simulink model "psbrectifier"  (Simulink 6.0)
settings: Solver=ode23tb  SolverMode=SingleTasking  StartTime=0.0  StopTime=0.1  RelTol=1e-3
libraries: powerlib2 x20
settings Model: Creator=patrice  LastModifiedBy=batserve  ExtModeTrigMode=oneshot  ExtModeArmWhenConnect=off  ExtModeAutoUpdateStatusClock=off
settings DataIOCC: LimitDataPoints=off  SignalLoggingName=sigsOut
settings OptimizationCC: BlockReduction=off  BooleanDataType=off
settings DebuggingCC: CheckExecutionContextPreStartOutputMsg=on  CheckExecutionContextRuntimeOutputMsg=on  SolverPrmCheckMsg=none
settings HardwareCC: TargetUnknown=on
settings RTWCC: TemplateMakefile=grt_unix.tmf

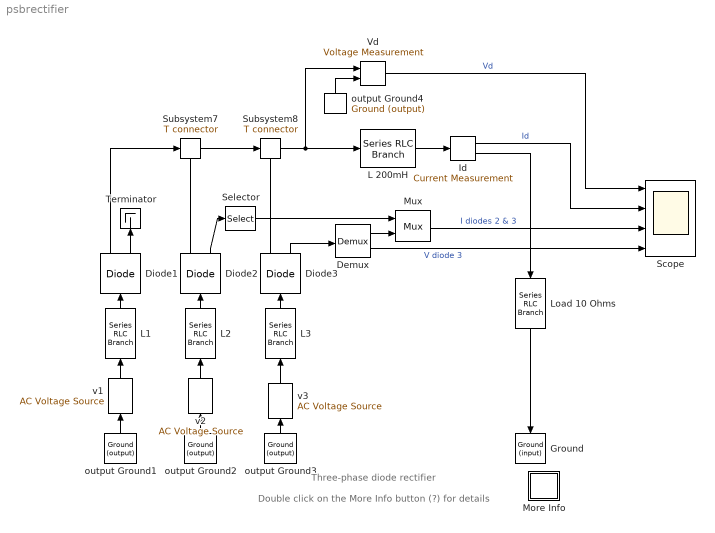
== system psbrectifier ==
  note: Double click on the More Info button (?) for details
  note: Three-phase diode rectifier
  Demux : Demux  Outputs=2
  Diode1 : powerlib2/Power Electronics/Diode  Tag=PoWeRsYsTeMbLoCk  Orientation=up  Ron=1e-2  Lon=0  Vf=0.8  IC=0  Rs=1000  Cs=0.1e-6  PSBOutputType=10
  Diode2 : powerlib2/Power Electronics/Diode  Tag=PoWeRsYsTeMbLoCk  Orientation=up  Ron=1e-2  Lon=0  Vf=0.8  IC=0  Rs=1000  Cs=0.1e-6  PSBOutputType=10
  Diode3 : powerlib2/Power Electronics/Diode  Tag=PoWeRsYsTeMbLoCk  Orientation=up  Ron=1e-2  Lon=0  Vf=0.8  IC=0  Rs=1000  Cs=0.1e-6  PSBOutputType=10
  Ground : powerlib2/Connectors/Ground (input)  Tag=PoWeRsYsTeMbLoCk  Orientation=down
  Id : powerlib2/Measurements/Current Measurement  Tag=PoWeRsYsTeMmEaSuReMeNt  PhasorSimulation=off  OutputType=Magnitude  PSBOutputType=01  PSBequivalent=0
  L 200mH : powerlib2/Elements/Series RLC Branch  Tag=PoWeRsYsTeMbLoCk  a=0  b=200e-03  c=inf  mesure=None  PSBOutputType=1
  L1 : powerlib2/Elements/Series RLC Branch  Tag=PoWeRsYsTeMbLoCk  Orientation=up  a=0  b=5e-03  c=inf  mesure=None  PSBOutputType=1
  L2 : powerlib2/Elements/Series RLC Branch  Tag=PoWeRsYsTeMbLoCk  Orientation=up  a=0  b=5e-03  c=inf  mesure=None  PSBOutputType=1
  L3 : powerlib2/Elements/Series RLC Branch  Tag=PoWeRsYsTeMbLoCk  Orientation=up  a=0  b=5e-03  c=inf  mesure=None  PSBOutputType=1
  Load 10 Ohms : powerlib2/Elements/Series RLC Branch  Tag=PoWeRsYsTeMbLoCk  Orientation=down  a=10  b=0  c=inf  mesure=None  PSBOutputType=1
  More Info : Subsystem
      mask Display: disp('?')
  Mux : Mux  Inputs=2
  Scope : Scope  NumInputPorts=4
      settings: TimeRange=0.1  YMin=0~0~0~-500  YMax=200~20~20~500  DataFormat=Structure
  Selector : Selector  Elements=1  InputPortWidth=2
  Subsystem7 : powerlib2/Connectors/T connector  Tag=PoWeRsYsTeMbLoCk  PSBOutputType=1
  Subsystem8 : powerlib2/Connectors/T connector  Tag=PoWeRsYsTeMbLoCk  PSBOutputType=1
  Terminator : Terminator
      settings: Orientation=up
  Vd : powerlib2/Measurements/Voltage Measurement  Tag=PoWeRsYsTeMmEaSuReMeNt  PhasorSimulation=off  OutputType=Magnitude  PSBOutputType=0  PSBequivalent=0
  output Ground{1..4} (4 alike) : powerlib2/Connectors/Ground (output)  Tag=PoWeRsYsTeMbLoCk  Orientation=up  PSBOutputType=1
  v1 : powerlib2/Electrical Sources/AC Voltage Source  Tag=PoWeRsYsTeMbLoCk  Orientation=up  A=120*sqrt(2)  P=0  F=60  stime=0  mesure=None  PSBOutputType=1
  v2 : powerlib2/Electrical Sources/AC Voltage Source  Tag=PoWeRsYsTeMbLoCk  Orientation=up  A=120*sqrt(2)  P=-120  F=60  stime=0  mesure=None  PSBOutputType=1
  v3 : powerlib2/Electrical Sources/AC Voltage Source  Tag=PoWeRsYsTeMbLoCk  Orientation=up  A=120*sqrt(2)  P=120  F=60  stime=0  mesure=None  PSBOutputType=1
  wires:
  Diode1/2 -> Terminator/1
  L 200mH/1 -> Id/1
  Id/2 -> Load 10 Ohms/1
  Load 10 Ohms/1 -> Ground/1
  output Ground1/1 -> v1/1
  L1/1 -> Diode1/1
  v1/1 -> L1/1
  output Ground2/1 -> v2/1
  L2/1 -> Diode2/1
  v2/1 -> L2/1
  output Ground3/1 -> v3/1
  L3/1 -> Diode3/1
  v3/1 -> L3/1
  Diode3/1 -> Subsystem8/Enable
  Subsystem7/1 -> Subsystem8/1
  Diode2/1 -> Subsystem7/Enable
  Diode1/1 -> Subsystem7/1
  Subsystem8/1 -> L 200mH/1, Vd/1
  output Ground4/1 -> Vd/2
  Selector/1 -> Mux/1
  Demux/1 -> Mux/2
  Diode2/2 -> Selector/1
  Diode3/2 -> Demux/1
  Vd/1 -> Scope/1  "Vd"
  Id/1 -> Scope/2  "Id"
  Mux/1 -> Scope/3  "I diodes 2 & 3"
  Demux/2 -> Scope/4  "V diode 3"

== system psbrectifier/More Info ==
  note: Demonstration
  note: Description
  note: This demonstration illustrates use of the Diode block
      | to simulate a three-phase rectifier and
      | compares continuous vs discrete simulations
  note: A 10 ohm load is fed in DC through a three-phase rectifier from an inductive
      | source (5 mH; 120 V rms). The rectified current is filtered by a 200mH inductance.
      |
      | Diodes are connected in parallel with RC snubbers (1000 ohms-0.1 uF)
      | The measurement outputs of Diode2 and  Diode3 is used to observe the diode voltage and current.
  note: 1. Simulation with continuous integration method
  note: 2. Simulation with discretized system
  note: Drag the 'Discrete system' block from the powerlib library into your psbrectifier system.
      | Keep the default sample time of 50 microseconds. Restart the simulation.
      |
      | Your system is now discretized and simulated at fixed time steps.
      | Compare  waveforms  with those obtained with the continuous integration algorithm (ode23tb).
  note: G. Sybille (Hydro-Quebec)
  note: Check  the simulation parameters in the Simulation/Parameters menu
      | The following intregation algorithm should be used: Variable time step ode23tb with default parameters.
      | Start the simulation and observe waveforms on the four trace Scope block.
      |
      | After a transient period the load current Id stabilizes at  12.7 A.  Note that  most of the  third harmonic which
      | can be seen in the rectified voltage Vd  (mean value 127 V) is filtered out by the  smoothing reactor.
      |
      | Observe also the commutation period  due to the source inductances.
      | The 3.3 degrees  overlap is clearly seen on  trace 3 of  the scope showing currents in  diodes 2 and 3.
      |
      | Zoom on the Diode3 voltage (trace 4)  during the conduction period. The voltage magnitude is the sum of the
      | specified  forward voltage (0.8 V) and the voltage developed  across the diode resistance (0.01 ohm).
